simulink model "L0203"  (R2015b)
settings: Solver=VariableStepAuto  StartTime=0.0  StopTime=100.0  MaxStep=0.01  RelTol=1e-3
libraries: simulink x2
settings Model: Creator=mmf.shpakAV  LastModifiedBy=mmf.shpakAV

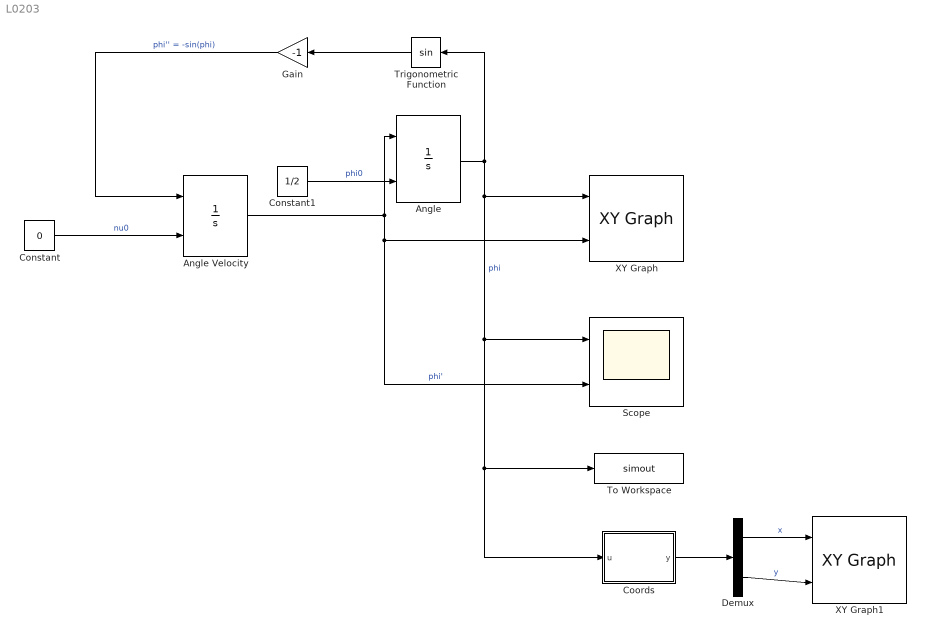
== system L0203 ==
  Angle : Integrator  InitialConditionSource=external
  Angle Velocity : Integrator  InitialConditionSource=external
  Constant : Constant  Value=0
  Constant1 : Constant  Value=1/2
  Coords : MATLAB Function  TreatAsAtomicUnit=on
  Demux : Demux  Outputs=2
  Gain : Gain  Gain=-1
  Scope : Scope  NumInputPorts=2
  To Workspace : ToWorkspace  VariableName=simout  SaveFormat=Structure With Time  SampleTime=-1
  Trigonometric Function : Trigonometry
  XY Graph : simulink/Sinks/XY Graph  xmin=-1  xmax=1  ymin=-1  ymax=1  st=-1
  XY Graph1 : simulink/Sinks/XY Graph  xmin=-1  xmax=1  ymin=-1  ymax=1  st=-1
  wires:
  Angle Velocity/1 -> Scope/2, XY Graph/2, Angle/1  "phi'"
  Angle/1 -> Scope/1, Coords/1(u), To Workspace/1, XY Graph/1, Trigonometric Function/1  "phi"
  Gain/1 -> Angle Velocity/1  "phi'' = -sin(phi)"
  Trigonometric Function/1 -> Gain/1
  Constant/1 -> Angle Velocity/2  "nu0"
  Constant1/1 -> Angle/2  "phi0"
  Demux/1 -> XY Graph1/1  "x"
  Demux/2 -> XY Graph1/2  "y"
  Coords/1(y) -> Demux/1

== matlab function L0203/Coords ==
  data: u input; y output
function y  = fcn(u)
%#codegen

y = [sin(u),-cos(u)]';
